simulink model "robotdynamic_simulink"  (R2018b)
settings: Solver=VariableStepAuto  StartTime=0.0  StopTime=10.0  RelTol=1e-3
values from neighbouring files (symbols this model uses):
  axel_len = .62    (= 0.62)    [controlWithLearnedSlipModel.m]    (also in run_model.m; wheelaccelDynamics.m)
settings Model: Creator=fworg  LastModifiedBy=fworg

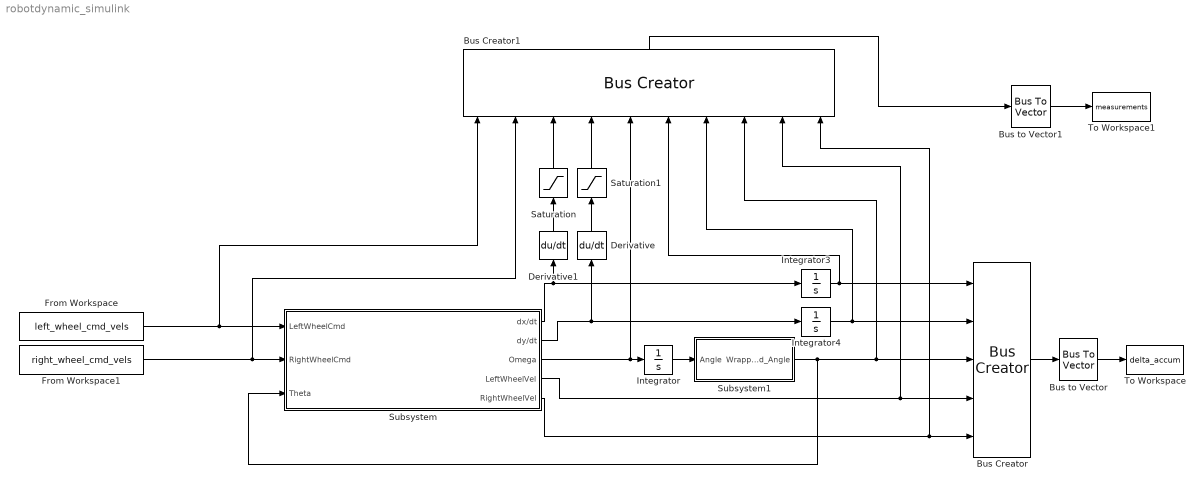
== system robotdynamic_simulink ==
  Bus Creator : BusCreator  Inputs=5
  Bus Creator1 : BusCreator  Inputs=10
  Bus to Vector : BusToVector
  Bus to Vector1 : BusToVector
  Derivative : Derivative
  Derivative1 : Derivative
  From Workspace : FromWorkspace  VariableName=left_wheel_cmd_vels  SampleTime=0  OutputAfterFinalValue=Setting to zero
  From Workspace1 : FromWorkspace  VariableName=right_wheel_cmd_vels  SampleTime=0  OutputAfterFinalValue=Setting to zero
  Integrator : Integrator
  Integrator3 : Integrator
  Integrator4 : Integrator
  Saturation : Saturate  UpperLimit=5  LowerLimit=-5
  Saturation1 : Saturate  UpperLimit=5  LowerLimit=-5
  Subsystem : Subsystem
  Subsystem1 : Subsystem
  To Workspace : ToWorkspace  VariableName=delta_accum  SaveFormat=Timeseries  SampleTime=-1
  To Workspace1 : ToWorkspace  VariableName=measurements  SaveFormat=Timeseries  SampleTime=-1
  wires:
  From Workspace1/1 -> Bus Creator1/2, Subsystem/2("RightWheelCmd ")
  From Workspace/1 -> Subsystem/1(LeftWheelCmd), Bus Creator1/1
  Subsystem/3(Omega) -> Bus Creator1/5, Integrator/1
  Subsystem/4(LeftWheelVel) -> Bus Creator/4, Bus Creator1/9
  Subsystem/5(RightWheelVel) -> Bus Creator/5, Bus Creator1/10
  Bus Creator/1 -> Bus to Vector/1
  Bus to Vector/1 -> To Workspace/1
  Integrator/1 -> Subsystem1/1(Angle)
  Subsystem1/1(Wrapped_Angle) -> Subsystem/3(Theta), Bus Creator/3, Bus Creator1/8
  Integrator4/1 -> Bus Creator/2, Bus Creator1/7
  Bus Creator1/1 -> Bus to Vector1/1
  Subsystem/1(dx/dt) -> Derivative1/1, Integrator3/1
  Subsystem/2(dy/dt) -> Derivative/1, Integrator4/1
  Integrator3/1 -> Bus Creator1/6, Bus Creator/1
  Bus to Vector1/1 -> To Workspace1/1
  Derivative/1 -> Saturation1/1
  Derivative1/1 -> Saturation/1
  Saturation/1 -> Bus Creator1/3
  Saturation1/1 -> Bus Creator1/4

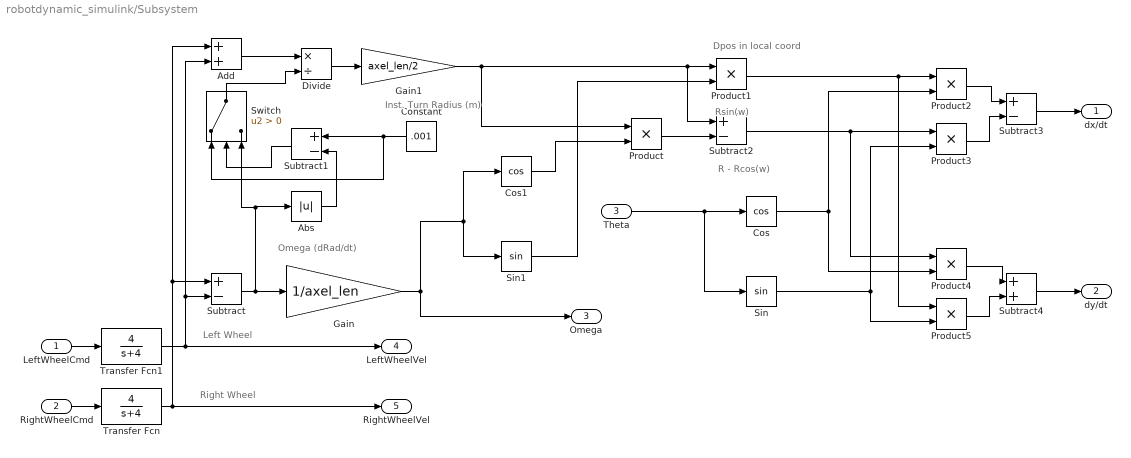
== system robotdynamic_simulink/Subsystem ==
  note: Rsin(w)
  note: R - Rcos(w)
  note: Dpos in local coord
  note: Right Wheel
  note: Left Wheel
  note: Omega (dRad/dt)
  note: Inst. Turn Radius (m)
  LeftWheelCmd : Inport
  "RightWheelCmd " : Inport  Port=2
  Theta : Inport  Port=3
  Abs : Abs
  Add : Sum
  Constant : Constant  Value=.001
  Cos : Trigonometry  Operator=cos
  Cos1 : Trigonometry  Operator=cos
  Divide : Product  Inputs=*/
  Gain : Gain  Gain=1/axel_len
  Gain1 : Gain  Gain=axel_len/2
  Product{,1..5} (6 alike) : Product
  Sin : Trigonometry
  Sin1 : Trigonometry
  Subtract{,1..3} (4 alike) : Sum  Inputs=+-
  Subtract4 : Sum
  Switch : Switch  Criteria=u2 > Threshold
  Transfer Fcn : TransferFcn  Numerator=[4]  Denominator=[1 4]  ContinuousStateAttributes='rightWheel'
  Transfer Fcn1 : TransferFcn  Numerator=[4]  Denominator=[1 4]  ContinuousStateAttributes='leftWheel'
  dx/dt : Outport
  dy/dt : Outport  Port=2
  Omega : Outport  Port=3
  LeftWheelVel : Outport  Port=4
  RightWheelVel : Outport  Port=5
  wires:
  "RightWheelCmd "/1 -> Transfer Fcn/1
  LeftWheelCmd/1 -> Transfer Fcn1/1
  Transfer Fcn1/1 -> LeftWheelVel/1, Add/2, Subtract/2
  Transfer Fcn/1 -> RightWheelVel/1, Add/1, Subtract/1
  Subtract/1 -> Abs/1, Switch/3, Gain/1
  Add/1 -> Divide/1
  Divide/1 -> Gain1/1
  Gain1/1 -> Product/1, Product1/1, Subtract2/1
  Cos1/1 -> Product/2
  Gain/1 -> Sin1/1, Cos1/1, Omega/1
  Sin1/1 -> Product1/2
  Switch/1 -> Divide/2
  Constant/1 -> Subtract1/1, Switch/1
  Subtract1/1 -> Switch/2
  Abs/1 -> Subtract1/2
  Product/1 -> Subtract2/2
  Theta/1 -> Sin/1, Cos/1
  Cos/1 -> Product2/2, Product4/2
  Sin/1 -> Product5/2, Product3/2
  Product1/1 -> Product2/1, Product5/1
  Product2/1 -> Subtract3/1
  Product3/1 -> Subtract3/2
  Product5/1 -> Subtract4/2
  Product4/1 -> Subtract4/1
  Subtract2/1 -> Product3/1, Product4/1
  Subtract3/1 -> dx/dt/1
  Subtract4/1 -> dy/dt/1

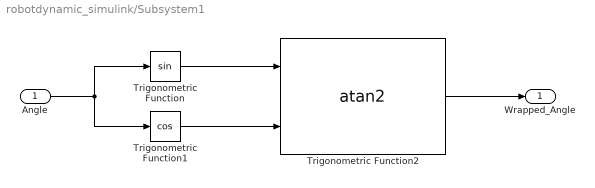
== system robotdynamic_simulink/Subsystem1 ==
  Angle : Inport
  Trigonometric Function : Trigonometry
  Trigonometric Function1 : Trigonometry  Operator=cos
  Trigonometric Function2 : Trigonometry  Operator=atan2
  Wrapped_Angle : Outport
  wires:
  Angle/1 -> Trigonometric Function1/1, Trigonometric Function/1
  Trigonometric Function1/1 -> Trigonometric Function2/2
  Trigonometric Function/1 -> Trigonometric Function2/1
  Trigonometric Function2/1 -> Wrapped_Angle/1
